simulink model "MLPQ4"  (R2022b)
settings: Solver=VariableStepAuto  StartTime=0.0  StopTime=2000  RelTol=1e-3
settings Model: Creator=Mojtaba  LastModifiedBy=AVAJANG
settings ModelReferenceCC: EnableRefExpFcnMdlSchedulingChecks=on

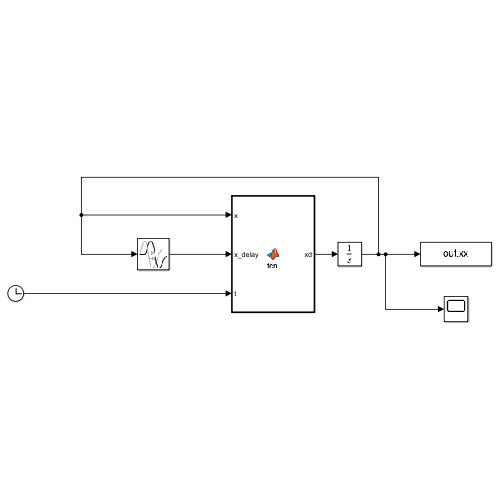
[thumbnail: Simulink's stored preview of the top-level diagram]
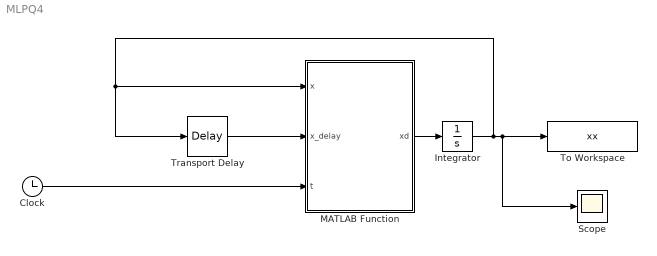
== system MLPQ4 ==
  Clock : Clock
  Integrator : Integrator  InitialCondition=1.2
  MATLAB Function : MATLAB Function  TreatAsAtomicUnit=on
  Scope : Scope
  To Workspace : ToWorkspace  VariableName=xx  SaveFormat=Timeseries  SampleTime=1
  Transport Delay : TransportDelay  DelayTime=17
  wires:
  MATLAB Function/1(xd) -> Integrator/1
  Integrator/1 -> MATLAB Function/1(x), Transport Delay/1, To Workspace/1, Scope/1
  Transport Delay/1 -> MATLAB Function/2(x_delay)
  Clock/1 -> MATLAB Function/3(t)

== matlab function MLPQ4/MATLAB Function ==
  data: x input; x_delay input; xd output; t input
function xd = fcn(x,x_delay,t)


tau=17;

if t-tau<0 
    xd=0;

elseif t-tau==0
   xd= (  (0.2*1.2)  /  (1+(1.2)^10)   )-0.1*x;

else
   xd= (  (0.2*x_delay)  /  (1+(x_delay)^10)   )-0.1*x;
end

end
